simulink model "sistemacomintegracao"  (R2020a)
settings: Solver=VariableStepAuto  StartTime=0.0  StopTime=10.0  RelTol=1e-3
values from neighbouring files (symbols this model uses):
  A = [[a11 a12];[a21 a22]]    [licao11.m]    (also in licao12.m = [[gamma 0]; [0 beta1]]; licao13_a.m = [0 1;0 -1]; licao13_ackerman.m = [-1.2 1;0 -0.8]; licao13_b.m = [1 T; 0 1])
  B = [epsilon; zeta]    [licao12.m]    (also in licao13_a.m = [0;10]; licao13_b.m = [0.5*T^2; T]; ordemreduzida.m = [0.00484; 0.0952]; projetolicao9.m = [0.002059 0.001686])
  C = [1 0]    [licao11a.m]    (also in licao12.m = [1 1]; licao13_a.m; ordemreduzida.m; provafinal.m = [-2 -3 2])
  K = [0 1]*inv([b A*b])*polyvalm(delta, A)    [licao13_ackerman.m]    (also in licao13_b.m = place(A,B,p); sistcomintegrador.m = place(A,B,[.9 .85 .8]))
  N = 100    [nyquist_livro.m]    (also in p1.m; sistcomintegrador.m = 0.1; transformada_z_classic.m = 15)
  Ts = 0.05    [licao9.m]    (also in licao9_controle.m; prova2b.m = 0.5; sistcomintegrador.m = 0.001)
settings Model: Creator=monica  LastModifiedBy=monica

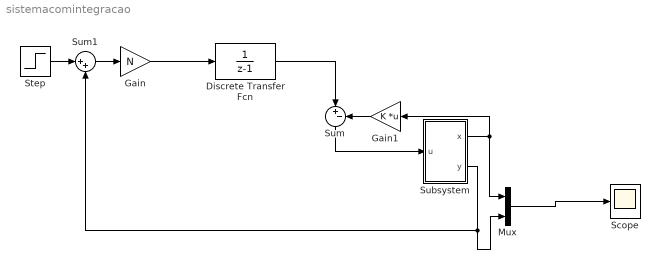
== system sistemacomintegracao ==
  Discrete Transfer Fcn : DiscreteTransferFcn  Denominator=[1 -1]  SampleTime=Ts
  Gain : Gain  Gain=N
  Gain1 : Gain  Gain=K  Multiplication=Matrix(K*u) (u vector)
  Mux : Mux  Inputs=2
  Scope : Scope
  Step : Step  SampleTime=0
  Subsystem : Subsystem
  Sum : Sum  Inputs=|+-
  Sum1 : Sum  Inputs=|++
  wires:
  Sum/1 -> Subsystem/1(u)
  Subsystem/1(x) -> Mux/1, Gain1/1
  Discrete Transfer Fcn/1 -> Sum/1
  Gain/1 -> Discrete Transfer Fcn/1
  Sum1/1 -> Gain/1
  Step/1 -> Sum1/1
  Gain1/1 -> Sum/2
  Subsystem/2(y) -> Mux/2, Sum1/2
  Mux/1 -> Scope/1

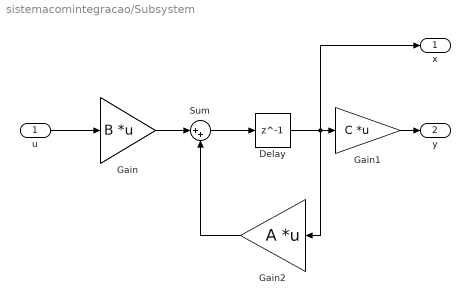
== system sistemacomintegracao/Subsystem ==
  u : Inport
  Delay : Delay  DelayLength=1  InitialCondition=0  SampleTime=Ts
  Gain : Gain  Gain=B  Multiplication=Matrix(K*u) (u vector)
  Gain1 : Gain  Gain=C  Multiplication=Matrix(K*u) (u vector)
  Gain2 : Gain  Gain=A  Multiplication=Matrix(K*u) (u vector)
  Sum : Sum  Inputs=|++
  x : Outport
  y : Outport  Port=2
  wires:
  Gain/1 -> Sum/1
  Delay/1 -> x/1, Gain2/1, Gain1/1
  Gain1/1 -> y/1
  Gain2/1 -> Sum/2
  u/1 -> Gain/1
  Sum/1 -> Delay/1
